simulink model "inductance"  (R2014a)
settings: Solver=ode45  StartTime=0.0  StopTime=10.0  RelTol=1e-3
values from neighbouring files (symbols this model uses):
  L0 = 0.0015    [tipe_vars.m]
  Lbob = 0.06    [tipe_vars.m]
libraries: simulink x1
settings Model: Creator=jackhalford  LastModifiedBy=jackhalford
settings SolverCC: ShapePreserveControl=EnableAll  ZeroCrossControl=DisableAll

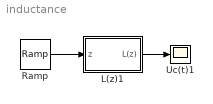
== system inductance ==
  L(z)1 : Subsystem
  Ramp : simulink/Sources/Ramp  slope=1  start=0  X0=0
  Uc(t)1 : Scope
      settings: ShowLegends=on  TimeRange=0.001  YMin=-800  YMax=-799.963  SaveName=ScopeData2
  wires:
  Ramp/1 -> L(z)1/1("z ")
  L(z)1/1(L(z)) -> Uc(t)1/1

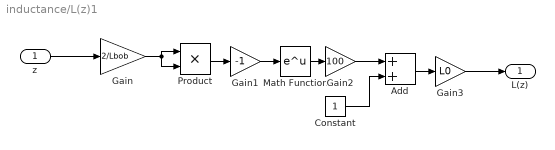
== system inductance/L(z)1 ==
  "z " : Inport
  Add : Sum
  Constant : Constant
  Gain : Gain  Gain=2/Lbob
  Gain1 : Gain  Gain=-1
  Gain2 : Gain  Gain=100
  Gain3 : Gain  Gain=L0
  Math Function : Math  SaturateOnIntegerOverflow=on
  Product : Product
  L(z) : Outport
  wires:
  "z "/1 -> Gain/1
  Gain/1 -> Product/1, Product/2
  Product/1 -> Gain1/1
  Gain1/1 -> Math Function/1
  Math Function/1 -> Gain2/1
  Gain2/1 -> Add/1
  Constant/1 -> Add/2
  Add/1 -> Gain3/1
  Gain3/1 -> L(z)/1
